simulink model "TST_EngDa_tiEngOn"  (R2016b)
settings: Solver=FixedStepDiscrete  StartTime=0.0  StopTime=7  FixedStep=sampleTime  RelTol=1e-3
values from neighbouring files (symbols this model uses):
  testCase = 1    [initTST_EngDa_tiEngOn_001.m]
libraries: simulink x3, UnitTest_Lib x1
settings Model: Creator=caijinkang  LastModifiedBy=caijinkang
settings DebuggingCC: SignalRangeChecking=error

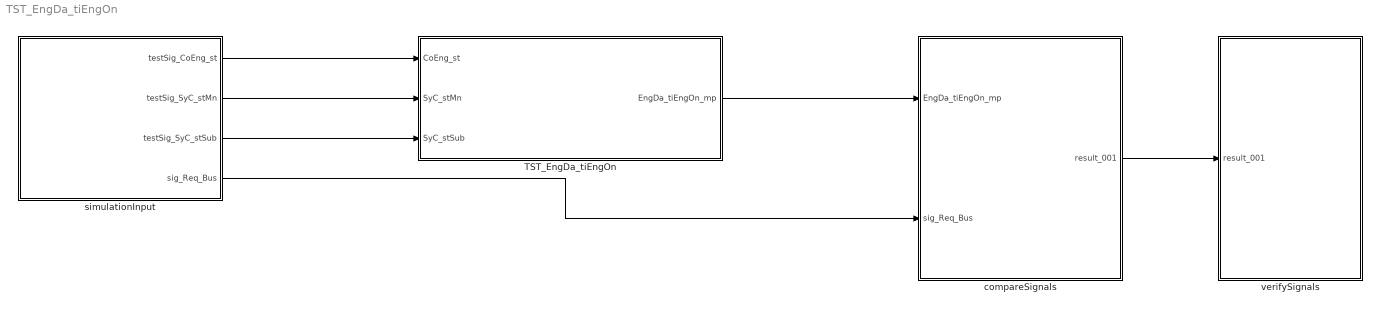
== system TST_EngDa_tiEngOn ==
  TST_EngDa_tiEngOn : Subsystem
  compareSignals : Subsystem
  simulationInput : Subsystem
  verifySignals : Subsystem
  wires:
  simulationInput/1(testSig_CoEng_st) -> TST_EngDa_tiEngOn/1(CoEng_st)
  simulationInput/2(testSig_SyC_stMn) -> TST_EngDa_tiEngOn/2(SyC_stMn)
  simulationInput/3(testSig_SyC_stSub) -> TST_EngDa_tiEngOn/3(SyC_stSub)
  TST_EngDa_tiEngOn/1(EngDa_tiEngOn_mp) -> compareSignals/1(EngDa_tiEngOn_mp)
  simulationInput/4(sig_Req_Bus) -> compareSignals/2(sig_Req_Bus)
  compareSignals/1(result_001) -> verifySignals/1(result_001)

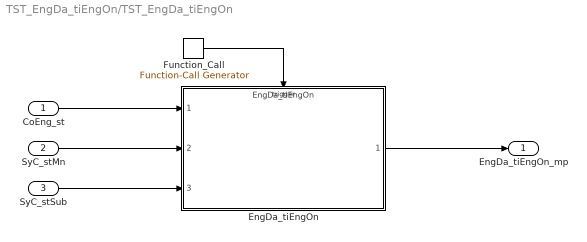
== system TST_EngDa_tiEngOn/TST_EngDa_tiEngOn ==
  CoEng_st : Inport
  SyC_stMn : Inport  Port=2
  SyC_stSub : Inport  Port=3
  EngDa_tiEngOn : ModelReference  ModelNameDialog=EngDa_tiEngOn  SimulationMode=Normal  ModelReferenceVersion=1.17  TriggerPortName=function  TriggerPortTriggerType=function-call  TriggerPortStatesWhenEnabling=held
  Function_Call : simulink/Ports & Subsystems/Function-Call Generator  sample_time=sampleTime  numberOfIterations=1
  EngDa_tiEngOn_mp : Outport
  wires:
  Function_Call/1 -> EngDa_tiEngOn/Trigger
  CoEng_st/1 -> EngDa_tiEngOn/1
  SyC_stMn/1 -> EngDa_tiEngOn/2
  SyC_stSub/1 -> EngDa_tiEngOn/3
  EngDa_tiEngOn/1 -> EngDa_tiEngOn_mp/1

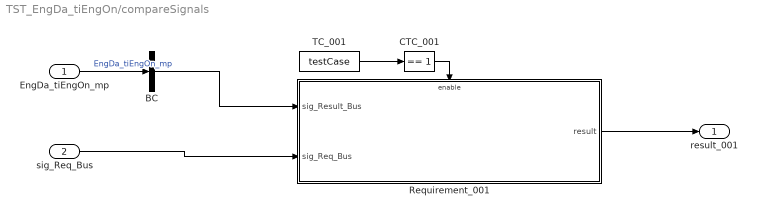
== system TST_EngDa_tiEngOn/compareSignals ==
  EngDa_tiEngOn_mp : Inport
  sig_Req_Bus : Inport  Port=2
  BC : BusCreator  Inputs=1
  CTC_001 : simulink/Logic and Bit Operations/Compare To Constant  relop===  const=1  OutDataTypeStr=boolean
  Requirement_001 : Subsystem
  TC_001 : Constant  Value=testCase
  result_001 : Outport
  wires:
  EngDa_tiEngOn_mp/1 -> BC/1  "EngDa_tiEngOn_mp"
  TC_001/1 -> CTC_001/1
  CTC_001/1 -> Requirement_001/Enable
  sig_Req_Bus/1 -> Requirement_001/2(sig_Req_Bus)
  BC/1 -> Requirement_001/1(sig_Result_Bus)
  Requirement_001/1(result) -> result_001/1

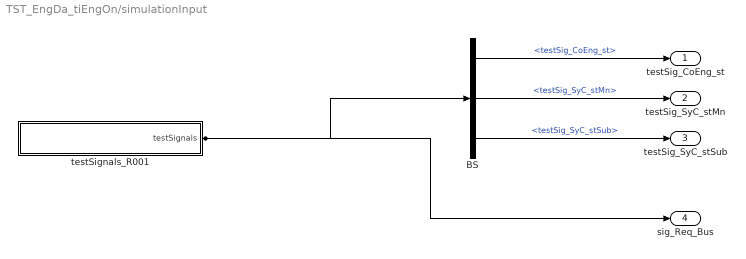
== system TST_EngDa_tiEngOn/simulationInput ==
  BS : BusSelector  OutputSignals=testSig_CoEng_st,testSig_SyC_stMn,testSig_SyC_stSub
  testSignals_R001 : Subsystem
  testSig_CoEng_st : Outport
  testSig_SyC_stMn : Outport  Port=2
  testSig_SyC_stSub : Outport  Port=3
  sig_Req_Bus : Outport  Port=4
  wires:
  BS/1 -> testSig_CoEng_st/1  "<testSig_CoEng_st>"
  BS/2 -> testSig_SyC_stMn/1  "<testSig_SyC_stMn>"
  BS/3 -> testSig_SyC_stSub/1  "<testSig_SyC_stSub>"
  testSignals_R001/1(testSignals) -> BS/1, sig_Req_Bus/1

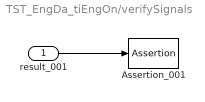
== system TST_EngDa_tiEngOn/verifySignals ==
  result_001 : Inport
  Assertion_001 : Assertion
  wires:
  result_001/1 -> Assertion_001/1

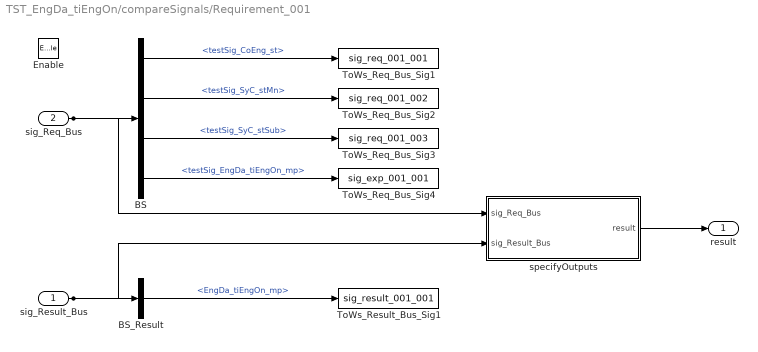
== system TST_EngDa_tiEngOn/compareSignals/Requirement_001 ==
  sig_Result_Bus : Inport
  sig_Req_Bus : Inport  Port=2
  Enable : EnablePort
  BS : BusSelector  OutputSignals=testSig_CoEng_st,testSig_SyC_stMn,testSig_SyC_stSub,testSig_EngDa_tiEngOn_mp
  BS_Result : BusSelector  OutputSignals=EngDa_tiEngOn_mp
  ToWs_Req_Bus_Sig1 : ToWorkspace  VariableName=sig_req_001_001  SaveFormat=Structure With Time
  ToWs_Req_Bus_Sig2 : ToWorkspace  VariableName=sig_req_001_002  SaveFormat=Structure With Time
  ToWs_Req_Bus_Sig3 : ToWorkspace  VariableName=sig_req_001_003  SaveFormat=Structure With Time
  ToWs_Req_Bus_Sig4 : ToWorkspace  VariableName=sig_exp_001_001  SaveFormat=Structure With Time
  ToWs_Result_Bus_Sig1 : ToWorkspace  VariableName=sig_result_001_001  SaveFormat=Structure With Time
  specifyOutputs : Subsystem
  result : Outport
  wires:
  sig_Req_Bus/1 -> BS/1, specifyOutputs/1(sig_Req_Bus)
  BS/1 -> ToWs_Req_Bus_Sig1/1  "<testSig_CoEng_st>"
  BS/2 -> ToWs_Req_Bus_Sig2/1  "<testSig_SyC_stMn>"
  BS/3 -> ToWs_Req_Bus_Sig3/1  "<testSig_SyC_stSub>"
  BS/4 -> ToWs_Req_Bus_Sig4/1  "<testSig_EngDa_tiEngOn_mp>"
  sig_Result_Bus/1 -> BS_Result/1, specifyOutputs/2(sig_Result_Bus)
  BS_Result/1 -> ToWs_Result_Bus_Sig1/1  "<EngDa_tiEngOn_mp>"
  specifyOutputs/1(result) -> result/1

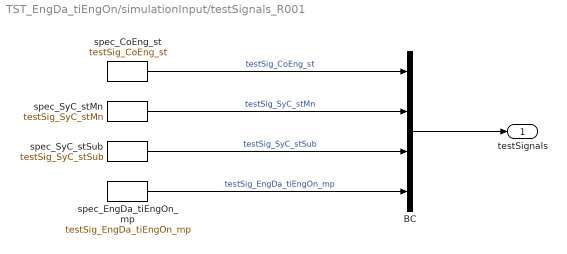
== system TST_EngDa_tiEngOn/simulationInput/testSignals_R001 ==
  BC : BusCreator  Inputs=4
  spec_CoEng_st : FromWorkspace  VariableName=testSig_CoEng_st  Interpolate=off  OutputAfterFinalValue=Holding final value
  spec_EngDa_tiEngOn_mp : FromWorkspace  VariableName=testSig_EngDa_tiEngOn_mp  Interpolate=off  OutputAfterFinalValue=Holding final value
  spec_SyC_stMn : FromWorkspace  VariableName=testSig_SyC_stMn  Interpolate=off  OutputAfterFinalValue=Holding final value
  spec_SyC_stSub : FromWorkspace  VariableName=testSig_SyC_stSub  Interpolate=off  OutputAfterFinalValue=Holding final value
  testSignals : Outport
  wires:
  BC/1 -> testSignals/1
  spec_CoEng_st/1 -> BC/1  "testSig_CoEng_st"
  spec_SyC_stMn/1 -> BC/2  "testSig_SyC_stMn"
  spec_SyC_stSub/1 -> BC/3  "testSig_SyC_stSub"
  spec_EngDa_tiEngOn_mp/1 -> BC/4  "testSig_EngDa_tiEngOn_mp"

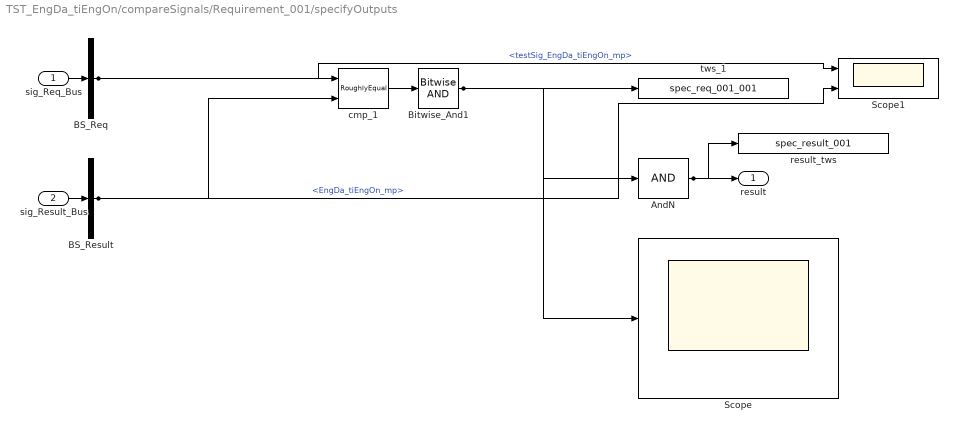
== system TST_EngDa_tiEngOn/compareSignals/Requirement_001/specifyOutputs ==
  sig_Req_Bus : Inport
  sig_Result_Bus : Inport  Port=2
  AndN : Logic  Inputs=1
  BS_Req : BusSelector  OutputSignals=testSig_EngDa_tiEngOn_mp
  BS_Result : BusSelector  OutputSignals=EngDa_tiEngOn_mp
  Bitwise_And1 : simulink/Logic and Bit Operations/Bitwise Operator  logicop=AND  UseBitMask=off  BitMask=bin2dec('11011001')  BitMaskRealWorld=Stored Integer
  Scope : Scope
  Scope1 : Scope  NumInputPorts=2
  cmp_1 : UnitTest_Lib/RoughlyEqual  slope=0.1
  result_tws : ToWorkspace  VariableName=spec_result_001
  tws_1 : ToWorkspace  VariableName=spec_req_001_001
  result : Outport
  wires:
  sig_Req_Bus/1 -> BS_Req/1
  sig_Result_Bus/1 -> BS_Result/1
  AndN/1 -> result/1, result_tws/1
  BS_Req/1 -> cmp_1/1, Scope1/1  "<testSig_EngDa_tiEngOn_mp>"
  BS_Result/1 -> cmp_1/2, Scope1/2  "<EngDa_tiEngOn_mp>"
  cmp_1/1 -> Bitwise_And1/1
  Bitwise_And1/1 -> tws_1/1, AndN/1, Scope/1
